simulink model "OLDip_RMS_testOLD"  (R2022b)
settings: Solver=FixedStepAuto  StartTime=0.0  StopTime=inf  FixedStep=Ts  RelTol=1e-3
undefined symbols (not defined in the file or in its folder): countsPerRev, maxPWM, motorN, pendDwnValue, Ts
libraries: arduinolib x6, slpidlib x3, arduinosensorlib x1, hdlsllib x1
settings Model: SimulationMode=external  ExtModeTrigDuration=2  Creator=47954  LastModifiedBy=47954
settings SolverCC: AutoInsertRateTranBlk=on
settings OptimizationCC: EnhancedBackFolding=on  PassReuseOutputArgsThreshold=0  MaxStackSize=64  OptimizeBlockOrder=speed  DifferentSizesBufferReuse=on  OptimizationCustomize=off
settings DebuggingCC: ParameterPrecisionLossMsg=none  ParameterTunabilityLossMsg=error
settings HardwareCC: ProdBitPerInt=16  ProdBitPerPointer=16  ProdBitPerSizeT=16  ProdBitPerPtrDiffT=16  ProdLargestAtomicFloat=None  ProdWordSize=8  ProdLongLongMode=on  ProdHWDeviceType=Atmel->AVR  UseEmbeddedCoderFeatures=off  UseSimulinkCoderFeatures=off
settings ModelReferenceCC: EnableRefExpFcnMdlSchedulingChecks=on
settings SFSimCC: MATLABDynamicMemAlloc=off
settings RTWCC: Description=Embedded Coder  SystemTargetFile=ert.tlc  HardwareBoard=Arduino Mega 2560  TemplateMakefile=ert_default_tmf  RTWVerbose=off  Toolchain=Arduino AVR
settings CodeAppCC: ForceParamTrailComments=on  OperatorAnnotations=on  MangleLength=10
settings ERTTargetCC: ERTCustomFileBanners=off  SupportContinuousTime=on  SupportNonInlinedSFcns=on  RemoveResetFunc=off  SupportVariableSizeSignals=on  ModelStepFunctionPrototypeControlCompliant=off  ExtMode=on  ExtModeTransport=3  ExtModeStaticAlloc=on  ExtModeStaticAllocSize=2048  ExtModeMexFile=ext_xcp  ExtModeMexArgs=0 6 921600  ExtModeIntrfLevel=Level2 - Open  ERTSrcFileBannerTemplate=codertarget_code_template.cgt  ERTHdrFileBannerTemplate=codertarget_code_template.cgt  ERTDataSrcFileTemplate=codertarget_code_template.cgt  ERTDataHdrFileTemplate=codertarget_code_template.cgt

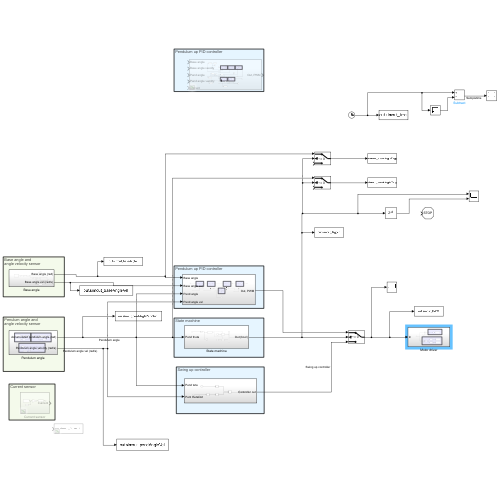
[thumbnail: Simulink's stored preview of the top-level diagram]
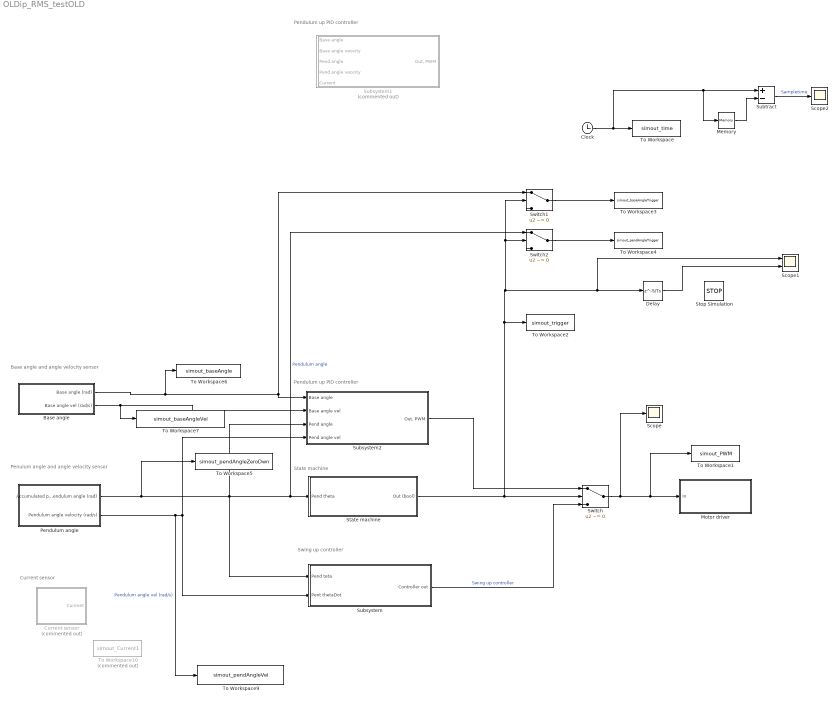
== system OLDip_RMS_testOLD ==
  note: State machine
  note: Swing up controller
  note: Penulum angle and
      | angle velocity sensor
  note: Base angle and
      | angle velocity sensor
  note: Current sensor
  note: Pendulum up PID controller
  note: Pendulum up PID controller
  Base angle : Subsystem
  Clock : Clock
  Current sensor : Subsystem  Commented=on
  Delay : Delay  DelayLength=5/Ts
  Memory : Memory
  Motor driver : Subsystem
  Pendulum angle : Subsystem
  Scope : Scope
  Scope1 : Scope  NumInputPorts=2
  Scope2 : Scope
  State machine : Subsystem
  Stop Simulation : Stop
  Subsystem : Subsystem
  Subsystem1 : Subsystem  Commented=on
  Subsystem2 : Subsystem
  Subtract : Sum  Inputs=+-
  Switch : Switch  Criteria=u2 ~= 0  SaturateOnIntegerOverflow=off  InputSameDT=off
  Switch1 : Switch  Criteria=u2 ~= 0  SaturateOnIntegerOverflow=off  InputSameDT=off
  Switch2 : Switch  Criteria=u2 ~= 0  SaturateOnIntegerOverflow=off  InputSameDT=off
  To Workspace : ToWorkspace  VariableName=simout_time  SampleTime=-1
      settings: Save2DSignal=2-D array (concatenate along first dimension)
  To Workspace1 : ToWorkspace  VariableName=simout_PWM  SampleTime=-1
      settings: Save2DSignal=2-D array (concatenate along first dimension)
  To Workspace10 : ToWorkspace  Commented=on  VariableName=simout_Current1  SampleTime=-1
      settings: Save2DSignal=2-D array (concatenate along first dimension)
  To Workspace2 : ToWorkspace  VariableName=simout_trigger  SampleTime=-1
      settings: Save2DSignal=2-D array (concatenate along first dimension)
  To Workspace3 : ToWorkspace  VariableName=simout_baseAngleTrigger  SampleTime=-1
      settings: Save2DSignal=2-D array (concatenate along first dimension)
  To Workspace4 : ToWorkspace  VariableName=simout_pendAngleTrigger  SampleTime=-1
      settings: Save2DSignal=2-D array (concatenate along first dimension)
  To Workspace5 : ToWorkspace  VariableName=simout_pendAngleZeroDwn  SampleTime=-1
      settings: Save2DSignal=2-D array (concatenate along first dimension)
  To Workspace6 : ToWorkspace  VariableName=simout_baseAngle  SampleTime=-1
      settings: Save2DSignal=2-D array (concatenate along first dimension)
  To Workspace7 : ToWorkspace  VariableName=simout_baseAngleVel  SampleTime=-1
      settings: Save2DSignal=2-D array (concatenate along first dimension)
  To Workspace9 : ToWorkspace  VariableName=simout_pendAngleVel  SampleTime=-1
      settings: Save2DSignal=2-D array (concatenate along first dimension)
  wires:
  Pendulum angle/1(Accumulated pendulum angle (rad)) -> To Workspace5/1, State machine/1(Pend theta), Switch2/1, Subsystem2/3(Pend angle), Subsystem/1(Pend teta)  "Pendulum angle"
  State machine/1(Out (bool)) -> Switch2/2, Switch1/2, Delay/1, Scope1/1, To Workspace2/1, Switch/2
  Subsystem/1(Controller out) -> Switch/3  "Swing up controller"
  Pendulum angle/2(Pendulum angle velocity (rad/s)) -> To Workspace9/1, Subsystem2/4(Pend angle vel), Subsystem/2(Pent thetaDot)  "Pendulum angle vel (rad/s)"
  Subsystem2/1("Out, PWM") -> Switch/1
  Base angle/1(Base angle (rad)) -> To Workspace6/1, Subsystem2/1(Base angle), Switch1/1
  Base angle/2(Base angle vel (rad/s)) -> To Workspace7/1, Subsystem2/2(Base angle vel)
  Switch/1 -> Scope/1, To Workspace1/1, Motor driver/1(In)
  Delay/1 -> Scope1/2
  Switch1/1 -> To Workspace3/1
  Switch2/1 -> To Workspace4/1
  Clock/1 -> Memory/1, Subtract/1, To Workspace/1
  Subtract/1 -> Scope2/1  "Sampletime"
  Memory/1 -> Subtract/2

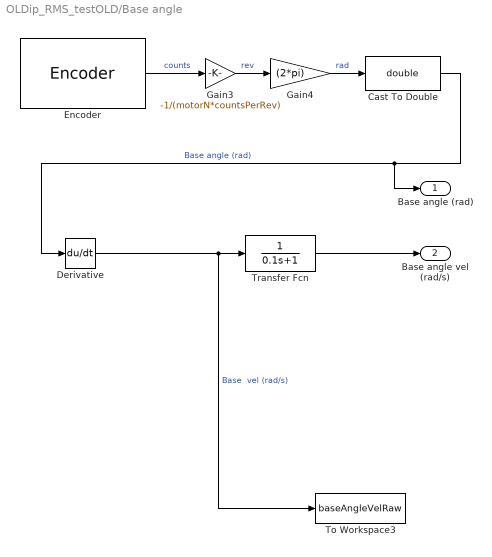
== system OLDip_RMS_testOLD/Base angle ==
  Cast To Double : DataTypeConversion  OutDataTypeStr=double  SaturateOnIntegerOverflow=off  RndMeth=Floor
  Derivative : Derivative
  Encoder : arduinosensorlib/Encoder  InputA=2  InputB=3  Mode=No reset  SampleTime=-1
  Gain3 : Gain  Gain=-1/(motorN*countsPerRev)
  Gain4 : Gain  Gain=(2*pi)
  To Workspace3 : ToWorkspace  VariableName=baseAngleVelRaw  SaveFormat=Structure With Time  SampleTime=-1
      settings: Save2DSignal=2-D array (concatenate along first dimension)
  Transfer Fcn : TransferFcn  Denominator=[0.1 1]
  Base angle (rad) : Outport
  Base angle vel (rad/s) : Outport  Port=2
  wires:
  Gain3/1 -> Gain4/1  "rev"
  Gain4/1 -> Cast To Double/1  "rad"
  Encoder/1 -> Gain3/1  "counts"
  Transfer Fcn/1 -> Base angle vel (rad/s)/1
  Derivative/1 -> To Workspace3/1, Transfer Fcn/1  "Base  vel (rad/s)"
  Cast To Double/1 -> Derivative/1, Base angle (rad)/1  "Base angle (rad)"

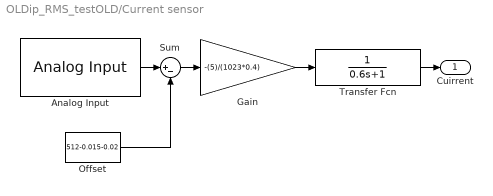
== system OLDip_RMS_testOLD/Current sensor ==
  Analog Input : arduinolib/Analog Input  pinNumber=10  ReadResultsOnly=off  ConversionTriggerSource=Software  ExternalTriggerType=uint32( 0 )  OutputDataType=uint16  EnableConversionCompleteNotify=off  EnableOuputStatus=off  SampleTime=-1  blockPlatform=arduino
  Gain : Gain  Gain=-(5)/(1023*0.4)
  Offset : Constant  Value=512-0.015-0.02
  Sum : Sum  Inputs=|+-
  Transfer Fcn : TransferFcn  Denominator=[0.6 1]
  Cuirrent : Outport
  wires:
  Offset/1 -> Sum/2
  Analog Input/1 -> Sum/1
  Gain/1 -> Transfer Fcn/1
  Transfer Fcn/1 -> Cuirrent/1
  Sum/1 -> Gain/1

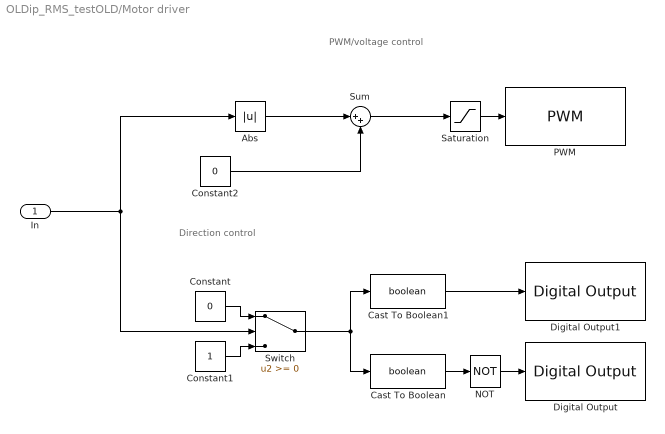
== system OLDip_RMS_testOLD/Motor driver ==
  note: PWM/voltage control
  note: Direction control
  In : Inport
  Abs : Abs  SaturateOnIntegerOverflow=off
  Cast To Boolean : DataTypeConversion  OutDataTypeStr=boolean  SaturateOnIntegerOverflow=off  RndMeth=Floor
  Cast To Boolean1 : DataTypeConversion  OutDataTypeStr=boolean  SaturateOnIntegerOverflow=off  RndMeth=Floor
  Constant : Constant  Value=0
  Constant1 : Constant
  Constant2 : Constant  Value=0
  Digital Output : arduinolib/Digital Output  pinNumber=4  Direction=output  blockPlatform=arduino
  Digital Output1 : arduinolib/Digital Output  pinNumber=5  Direction=output  blockPlatform=arduino
  NOT : Logic  Operator=NOT  IconShape=distinctive  AllPortsSameDT=off  OutDataTypeStr=boolean
  PWM : arduinolib/PWM  pinNumber=13  frequencyType=Specify  desiredFrequency=490.2*2  achievableFrequency=980.4
  Saturation : Saturate  UpperLimit=maxPWM  LowerLimit=-maxPWM
  Sum : Sum  Inputs=|++
  Switch : Switch  SaturateOnIntegerOverflow=off  InputSameDT=off
  wires:
  Constant1/1 -> Switch/3
  Cast To Boolean1/1 -> Digital Output1/1
  Constant/1 -> Switch/1
  In/1 -> Switch/2, Abs/1
  Switch/1 -> Cast To Boolean/1, Cast To Boolean1/1
  Cast To Boolean/1 -> NOT/1
  NOT/1 -> Digital Output/1
  Saturation/1 -> PWM/1
  Abs/1 -> Sum/1
  Sum/1 -> Saturation/1
  Constant2/1 -> Sum/2

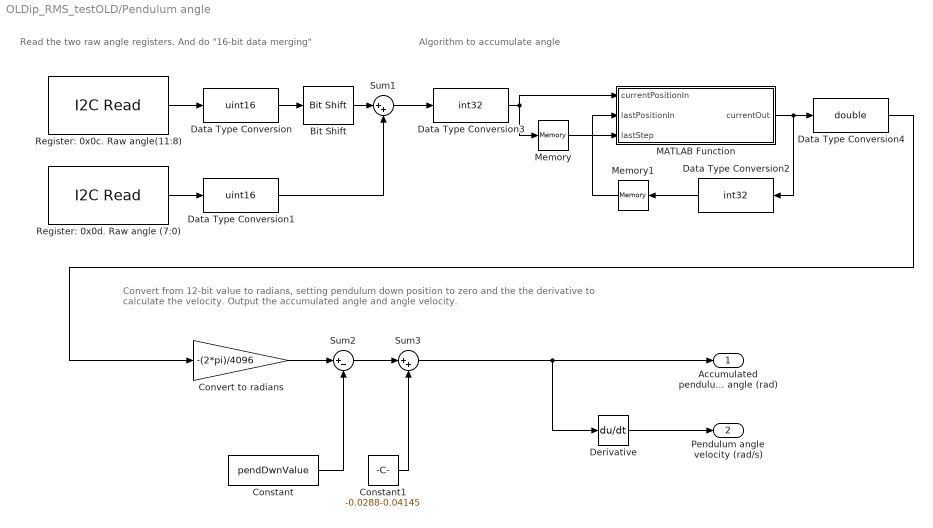
== system OLDip_RMS_testOLD/Pendulum angle ==
  note: Algorithm to accumulate angle
  note: Read the two raw angle registers.
      | And do "16-bit data merging"
  note: Convert from 12-bit value to radians, setting pendulum down position to zero and the the derivative
      | to calculate the velocity. Output the accumulated angle and angle velocity.
  Bit Shift : hdlsllib/Logic and Bit Operations/Bit Shift  mode=Shift Left Logical  N=8
  Constant : Constant  Value=pendDwnValue
  Constant1 : Constant  Value=-0.0288-0.04145
  Convert to radians : Gain  Gain=-(2*pi)/4096
  Data Type Conversion : DataTypeConversion  OutDataTypeStr=uint16  SaturateOnIntegerOverflow=off  RndMeth=Floor
  Data Type Conversion1 : DataTypeConversion  OutDataTypeStr=uint16  SaturateOnIntegerOverflow=off  RndMeth=Floor
  Data Type Conversion2 : DataTypeConversion  OutDataTypeStr=int32  SaturateOnIntegerOverflow=off  RndMeth=Floor
  Data Type Conversion3 : DataTypeConversion  OutDataTypeStr=int32  SaturateOnIntegerOverflow=off  RndMeth=Floor
  Data Type Conversion4 : DataTypeConversion  OutDataTypeStr=double  SaturateOnIntegerOverflow=off  RndMeth=Floor
  Derivative : Derivative
  "MATLAB Function " : MATLAB Function  TreatAsAtomicUnit=on
  Memory : Memory
  Memory1 : Memory
  Register: 0x0c. Raw angle(11:8) : arduinolib/I2C Read  I2CModule=0  Mode=Master  SlaveAddress=0x36  SlaveByteOrder=BigEndian  Direction=Receiver  RegisterAddressMode=on  RegisterAddress=0x0c  SlaveDataType=uint8  DataLength=1  NoAck=off  RepeatedStart=off  OutputStatus=off  blockPlatform=ARDUINO  SampleTime=-1
  Register: 0x0d. Raw angle (7:0) : arduinolib/I2C Read  I2CModule=0  Mode=Master  SlaveAddress=0x36  SlaveByteOrder=BigEndian  Direction=Receiver  RegisterAddressMode=on  RegisterAddress=0x0d  SlaveDataType=uint8  DataLength=1  NoAck=off  RepeatedStart=off  OutputStatus=off  blockPlatform=ARDUINO  SampleTime=-1
  Sum1 : Sum  Inputs=|++
  Sum2 : Sum  Inputs=|+-
  Sum3 : Sum  Inputs=|++
  Accumulated pendulum angle (rad) : Outport
  Pendulum angle velocity (rad/s) : Outport  Port=2
  wires:
  Memory/1 -> "MATLAB Function "/3(lastStep)
  Register: 0x0c. Raw angle(11:8)/1 -> Data Type Conversion/1
  Data Type Conversion3/1 -> Memory/1, "MATLAB Function "/1(currentPositionIn)
  Sum1/1 -> Data Type Conversion3/1
  Register: 0x0d. Raw angle (7:0)/1 -> Data Type Conversion1/1
  Bit Shift/1 -> Sum1/1
  Memory1/1 -> "MATLAB Function "/2(lastPositionIn)
  Data Type Conversion1/1 -> Sum1/2
  Data Type Conversion/1 -> Bit Shift/1
  "MATLAB Function "/1(currentOut) -> Data Type Conversion4/1, Data Type Conversion2/1
  Data Type Conversion2/1 -> Memory1/1
  Data Type Conversion4/1 -> Convert to radians/1
  Convert to radians/1 -> Sum2/1
  Sum3/1 -> Accumulated pendulum angle (rad)/1, Derivative/1
  Derivative/1 -> Pendulum angle velocity (rad/s)/1
  Constant/1 -> Sum2/2
  Constant1/1 -> Sum3/2
  Sum2/1 -> Sum3/1

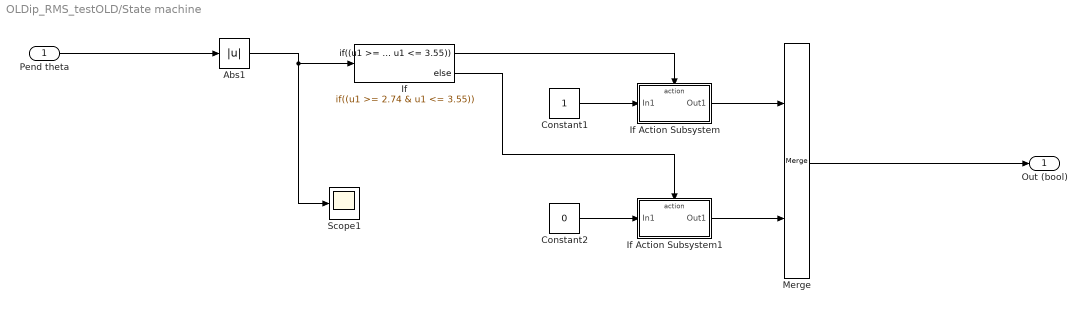
== system OLDip_RMS_testOLD/State machine ==
  Pend theta : Inport
  Abs1 : Abs  SaturateOnIntegerOverflow=off
  Constant1 : Constant
  Constant2 : Constant  Value=0
  If : If  IfExpression=(u1 >= 2.74 & u1 <= 3.55)
  If Action Subsystem : Subsystem  TreatAsAtomicUnit=on
  If Action Subsystem1 : Subsystem  TreatAsAtomicUnit=on
  Merge : Merge
  Scope1 : Scope
  Out (bool) : Outport
  wires:
  Constant1/1 -> If Action Subsystem/1(In1)
  If Action Subsystem/1(Out1) -> Merge/1
  If/1 -> If Action Subsystem/Action
  Pend theta/1 -> Abs1/1
  If/2 -> If Action Subsystem1/Action
  If Action Subsystem1/1(Out1) -> Merge/2
  Constant2/1 -> If Action Subsystem1/1(In1)
  Abs1/1 -> Scope1/1, If/1
  Merge/1 -> Out (bool)/1

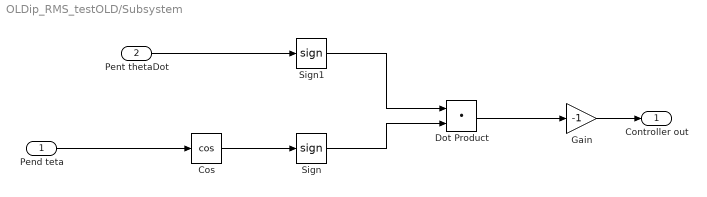
== system OLDip_RMS_testOLD/Subsystem ==
  Pend teta : Inport
  Pent thetaDot : Inport  Port=2
  Cos : Trigonometry  Operator=cos
  Dot Product : DotProduct  OutDataTypeStr=Inherit: Inherit via internal rule
  Gain : Gain  Gain=-1
  Sign : Signum
  Sign1 : Signum
  Controller out : Outport
  wires:
  Pend teta/1 -> Cos/1
  Sign1/1 -> Dot Product/1
  Pent thetaDot/1 -> Sign1/1
  Dot Product/1 -> Gain/1
  Sign/1 -> Dot Product/2
  Cos/1 -> Sign/1
  Gain/1 -> Controller out/1

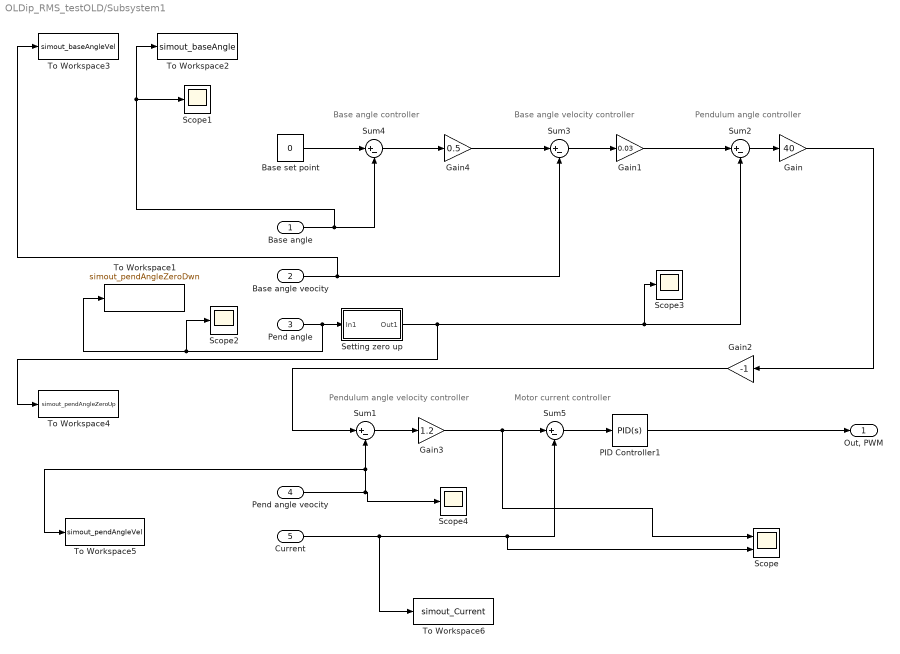
== system OLDip_RMS_testOLD/Subsystem1 ==
  note: Pendulum angle velocity controller
  note: Pendulum angle controller
  note: Base angle velocity controller
  note: Base angle controller
  note: Motor current controller
  Base angle : Inport
  Base angle veocity : Inport  Port=2
  Pend angle : Inport  Port=3
  Pend angle veocity : Inport  Port=4
  Current : Inport  Port=5
  Base set point : Constant  Value=0
  Gain : Gain  Gain=40
  Gain1 : Gain  Gain=0.03
  Gain2 : Gain  Gain=-1
  Gain3 : Gain  Gain=1.2
  Gain4 : Gain  Gain=0.5
  PID Controller1 : slpidlib/PID Controller  Controller=PID  Form=Parallel  TimeDomain=Continuous-time  UseExternalTs=off  SampleTime=-1  IntegratorMethod=Forward Euler  FilterMethod=Forward Euler  ControllerParametersSource=internal  P=30  I=0  UseKiTs=off  D=0  N=100  UseFilter=on  TunerSelectOption=Transfer Function Based (PID Tuner App)  InitialConditionSource=internal  InitialConditionForIntegrator=0  InitialConditionForFilter=0  DifferentiatorICPrevScaledInput=0  ExternalReset=none  TrackingMode=off  Kt=1  LimitOutput=off  SatLimitsSource=internal  UpperSaturationLimit=6  LowerSaturationLimit=-6  LinearizeAsGain=on  AntiWindupMode=clamping  Kb=1  LimitIntegrator=off  UpperIntegratorSaturationLimit=inf  LowerIntegratorSaturationLimit=-inf  POutMin=[]  POutMax=[]  IOutMin=[]  IOutMax=[]  DOutMin=[]  DOutMax=[]  NOutMin=[]  NOutMax=[]  SumOutMin=[]  SumOutMax=[]  SaturationOutMin=[]  SaturationOutMax=[]  PParamMin=[]  PParamMax=[]  IParamMin=[]  IParamMax=[]  DParamMin=[]  DParamMax=[]  NParamMin=[]  NParamMax=[]  KbParamMin=[]  KbParamMax=[]  KtParamMin=[]  KtParamMax=[]  KbOutMin=[]  KbOutMax=[]  KtOutMin=[]  KtOutMax=[]  IntegratorOutMin=[]  IntegratorOutMax=[]  FilterOutMin=[]  FilterOutMax=[]  SumI1OutMin=[]  SumI1OutMax=[]  SumI2OutMin=[]  SumI2OutMax=[]  SumI3OutMin=[]  SumI3OutMax=[]  SumI4OutMin=[]  SumI4OutMax=[]  SumDOutMin=[]  SumDOutMax=[]  DifferentiatorOutMin=[]  DifferentiatorOutMax=[]  FilterDiffOutCoefMin=[]  FilterDiffOutCoefMax=[]  ReciprocalOutMin=[]  ReciprocalOutMax=[]  SumDenOutMin=[]  SumDenOutMax=[]  SumNumOutMin=[]  SumNumOutMax=[]  DivideOutMin=[]  DivideOutMax=[]  UdiffTsProdOutMin=[]  UdiffTsProdOutMax=[]  NTsProdOutMin=[]  NTsProdOutMax=[]  UintegralTsProdOutMin=[]  UintegralTsProdOutMax=[]  UngainTsProdOutMin=[]  UngainTsProdOutMax=[]  ClampingZeroOutDataTypeStr=Inherit: Inherit via back propagation  ClampingZeroOutMin=[]  ClampingZeroOutMax=[]  FilterDenConstantOutDataTypeStr=Inherit: Inherit via back propagation  FilterDenConstantOutMin=[]  FilterDenConstantOutMax=[]  PCopyOutDataTypeStr=Inherit: Inherit via back propagation  PCopyOutMin=[]  PCopyOutMax=[]  NCopyOutDataTypeStr=Inherit: Inherit via back propagation  NCopyOutMin=[]  NCopyOutMax=[]  IntegratorContinuousStateAttributes=''  IntegratorStateMustResolveToSignalObject=off  IntegratorRTWStateStorageClass=Auto  FilterContinuousStateAttributes=''  FilterStateMustResolveToSignalObject=off  FilterRTWStateStorageClass=Auto  ParallelPVariant=InternalParameters  IdealPVariant=Disabled  IVariant=InternalParameters  DVariant=InternalParameters  IntegratorVariant=Continuous  SatVariant=Disabled  AWVariant=Passthrough  PCopyVariant=Disabled  TRVariant=Disabled  FdbkBlocksVariant=Forward  IdealPFdbkVariant=Disabled  SatFdbkVariant=Disabled  DerivativeFilterVariant=ContFilter  NVariant=InternalParameters  NCopyVariant=Disabled  FilterICVariant=InternalICsFilter  IntegratorICVariant=InternalICs  ExternalResetVariant=Disabled  TRSumVariant=Passthrough  SumFdbkVariant=Disabled  SumVariant=Sum_PID  TsampFilterVariant=InternalTs  TsampNgainVariant=Passthrough  TsampIntegralVariant=Passthrough  ExternalSaturationOutDataTypeStr=Inherit: Same as second input
  Scope : Scope  NumInputPorts=2
  Scope{1..4} (4 alike) : Scope
  "Setting zero up " : Subsystem
  Sum{1..5} (5 alike) : Sum  Inputs=|+-
  To Workspace1 : ToWorkspace  VariableName=simout_pendAngleZeroDwn  SampleTime=-1
      settings: Save2DSignal=2-D array (concatenate along first dimension)
  To Workspace2 : ToWorkspace  VariableName=simout_baseAngle  SampleTime=-1
      settings: Save2DSignal=2-D array (concatenate along first dimension)
  To Workspace3 : ToWorkspace  VariableName=simout_baseAngleVel  SampleTime=-1
      settings: Save2DSignal=2-D array (concatenate along first dimension)
  To Workspace4 : ToWorkspace  VariableName=simout_pendAngleZeroUp  SampleTime=-1
      settings: Save2DSignal=2-D array (concatenate along first dimension)
  To Workspace5 : ToWorkspace  VariableName=simout_pendAngleVel  SampleTime=-1
      settings: Save2DSignal=2-D array (concatenate along first dimension)
  To Workspace6 : ToWorkspace  VariableName=simout_Current  SampleTime=-1
      settings: Save2DSignal=2-D array (concatenate along first dimension)
  "Out, PWM" : Outport
  wires:
  Sum2/1 -> Gain/1
  Sum1/1 -> Gain3/1
  Gain/1 -> Gain2/1
  Pend angle veocity/1 -> Scope4/1, To Workspace5/1, Sum1/2
  Sum4/1 -> Gain4/1
  Sum3/1 -> Gain1/1
  Gain1/1 -> Sum2/1
  Gain2/1 -> Sum1/1
  Base angle/1 -> Scope1/1, To Workspace2/1, Sum4/2
  Gain4/1 -> Sum3/1
  Base set point/1 -> Sum4/1
  Sum5/1 -> PID Controller1/1
  Gain3/1 -> Scope/1, Sum5/1
  PID Controller1/1 -> "Out, PWM"/1
  Current/1 -> To Workspace6/1, Scope/2, Sum5/2
  Pend angle/1 -> Scope2/1, To Workspace1/1, "Setting zero up "/1(In1)
  "Setting zero up "/1(Out1) -> To Workspace4/1, Scope3/1, Sum2/2
  Base angle veocity/1 -> To Workspace3/1, Sum3/2

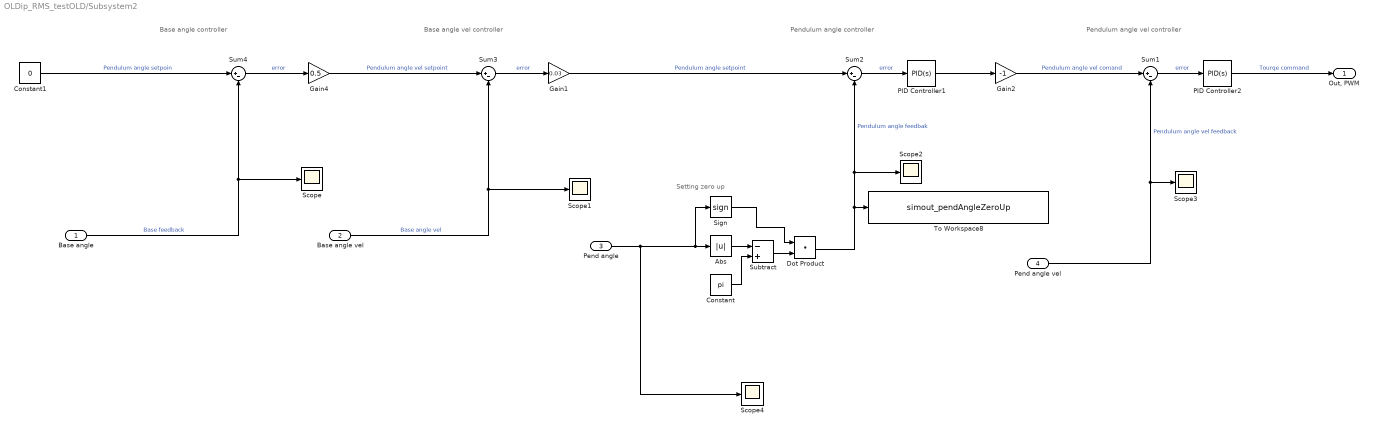
== system OLDip_RMS_testOLD/Subsystem2 ==
  note: Setting zero up
  note: Pendulum angle controller
  note: Pendulum angle vel controller
  note: Base angle vel controller
  note: Base angle controller
  Base angle : Inport
  Base angle vel : Inport  Port=2
  Pend angle : Inport  Port=3
  Pend angle vel : Inport  Port=4
  Abs : Abs  SaturateOnIntegerOverflow=off
  Constant : Constant  Value=pi
  Constant1 : Constant  Value=0
  Dot Product : DotProduct  OutDataTypeStr=Inherit: Inherit via internal rule
  Gain1 : Gain  Gain=0.03
  Gain2 : Gain  Gain=-1
  Gain4 : Gain  Gain=0.5
  PID Controller1 : slpidlib/PID Controller  Controller=PID  Form=Parallel  TimeDomain=Continuous-time  UseExternalTs=off  SampleTime=-1  IntegratorMethod=Forward Euler  FilterMethod=Forward Euler  ControllerParametersSource=internal  P=45  I=0  UseKiTs=off  D=0  N=100  UseFilter=on  TunerSelectOption=Transfer Function Based (PID Tuner App)  InitialConditionSource=internal  InitialConditionForIntegrator=0  InitialConditionForFilter=0  DifferentiatorICPrevScaledInput=0  ExternalReset=none  TrackingMode=off  Kt=1  LimitOutput=off  SatLimitsSource=internal  UpperSaturationLimit=6  LowerSaturationLimit=-6  LinearizeAsGain=on  AntiWindupMode=clamping  Kb=1  LimitIntegrator=off  UpperIntegratorSaturationLimit=inf  LowerIntegratorSaturationLimit=-inf  POutMin=[]  POutMax=[]  IOutMin=[]  IOutMax=[]  DOutMin=[]  DOutMax=[]  NOutMin=[]  NOutMax=[]  SumOutMin=[]  SumOutMax=[]  SaturationOutMin=[]  SaturationOutMax=[]  PParamMin=[]  PParamMax=[]  IParamMin=[]  IParamMax=[]  DParamMin=[]  DParamMax=[]  NParamMin=[]  NParamMax=[]  KbParamMin=[]  KbParamMax=[]  KtParamMin=[]  KtParamMax=[]  KbOutMin=[]  KbOutMax=[]  KtOutMin=[]  KtOutMax=[]  IntegratorOutMin=[]  IntegratorOutMax=[]  FilterOutMin=[]  FilterOutMax=[]  SumI1OutMin=[]  SumI1OutMax=[]  SumI2OutMin=[]  SumI2OutMax=[]  SumI3OutMin=[]  SumI3OutMax=[]  SumI4OutMin=[]  SumI4OutMax=[]  SumDOutMin=[]  SumDOutMax=[]  DifferentiatorOutMin=[]  DifferentiatorOutMax=[]  FilterDiffOutCoefMin=[]  FilterDiffOutCoefMax=[]  ReciprocalOutMin=[]  ReciprocalOutMax=[]  SumDenOutMin=[]  SumDenOutMax=[]  SumNumOutMin=[]  SumNumOutMax=[]  DivideOutMin=[]  DivideOutMax=[]  UdiffTsProdOutMin=[]  UdiffTsProdOutMax=[]  NTsProdOutMin=[]  NTsProdOutMax=[]  UintegralTsProdOutMin=[]  UintegralTsProdOutMax=[]  UngainTsProdOutMin=[]  UngainTsProdOutMax=[]  ClampingZeroOutDataTypeStr=Inherit: Inherit via back propagation  ClampingZeroOutMin=[]  ClampingZeroOutMax=[]  FilterDenConstantOutDataTypeStr=Inherit: Inherit via back propagation  FilterDenConstantOutMin=[]  FilterDenConstantOutMax=[]  PCopyOutDataTypeStr=Inherit: Inherit via back propagation  PCopyOutMin=[]  PCopyOutMax=[]  NCopyOutDataTypeStr=Inherit: Inherit via back propagation  NCopyOutMin=[]  NCopyOutMax=[]  IntegratorContinuousStateAttributes=''  IntegratorStateMustResolveToSignalObject=off  IntegratorRTWStateStorageClass=Auto  FilterContinuousStateAttributes=''  FilterStateMustResolveToSignalObject=off  FilterRTWStateStorageClass=Auto  ParallelPVariant=InternalParameters  IdealPVariant=Disabled  IVariant=InternalParameters  DVariant=InternalParameters  IntegratorVariant=Continuous  SatVariant=Disabled  AWVariant=Passthrough  PCopyVariant=Disabled  TRVariant=Disabled  FdbkBlocksVariant=Forward  IdealPFdbkVariant=Disabled  SatFdbkVariant=Disabled  DerivativeFilterVariant=ContFilter  NVariant=InternalParameters  NCopyVariant=Disabled  FilterICVariant=InternalICsFilter  IntegratorICVariant=InternalICs  ExternalResetVariant=Disabled  TRSumVariant=Passthrough  SumFdbkVariant=Disabled  SumVariant=Sum_PID  TsampFilterVariant=InternalTs  TsampNgainVariant=Passthrough  TsampIntegralVariant=Passthrough  ExternalSaturationOutDataTypeStr=Inherit: Same as second input
  PID Controller2 : slpidlib/PID Controller  Controller=PID  Form=Parallel  TimeDomain=Continuous-time  UseExternalTs=off  SampleTime=-1  IntegratorMethod=Forward Euler  FilterMethod=Forward Euler  ControllerParametersSource=internal  P=45  I=0  UseKiTs=off  D=0  N=100  UseFilter=on  TunerSelectOption=Transfer Function Based (PID Tuner App)  InitialConditionSource=internal  InitialConditionForIntegrator=0  InitialConditionForFilter=0  DifferentiatorICPrevScaledInput=0  ExternalReset=none  TrackingMode=off  Kt=1  LimitOutput=off  SatLimitsSource=internal  UpperSaturationLimit=6  LowerSaturationLimit=-6  LinearizeAsGain=on  AntiWindupMode=clamping  Kb=1  LimitIntegrator=off  UpperIntegratorSaturationLimit=inf  LowerIntegratorSaturationLimit=-inf  POutMin=[]  POutMax=[]  IOutMin=[]  IOutMax=[]  DOutMin=[]  DOutMax=[]  NOutMin=[]  NOutMax=[]  SumOutMin=[]  SumOutMax=[]  SaturationOutMin=[]  SaturationOutMax=[]  PParamMin=[]  PParamMax=[]  IParamMin=[]  IParamMax=[]  DParamMin=[]  DParamMax=[]  NParamMin=[]  NParamMax=[]  KbParamMin=[]  KbParamMax=[]  KtParamMin=[]  KtParamMax=[]  KbOutMin=[]  KbOutMax=[]  KtOutMin=[]  KtOutMax=[]  IntegratorOutMin=[]  IntegratorOutMax=[]  FilterOutMin=[]  FilterOutMax=[]  SumI1OutMin=[]  SumI1OutMax=[]  SumI2OutMin=[]  SumI2OutMax=[]  SumI3OutMin=[]  SumI3OutMax=[]  SumI4OutMin=[]  SumI4OutMax=[]  SumDOutMin=[]  SumDOutMax=[]  DifferentiatorOutMin=[]  DifferentiatorOutMax=[]  FilterDiffOutCoefMin=[]  FilterDiffOutCoefMax=[]  ReciprocalOutMin=[]  ReciprocalOutMax=[]  SumDenOutMin=[]  SumDenOutMax=[]  SumNumOutMin=[]  SumNumOutMax=[]  DivideOutMin=[]  DivideOutMax=[]  UdiffTsProdOutMin=[]  UdiffTsProdOutMax=[]  NTsProdOutMin=[]  NTsProdOutMax=[]  UintegralTsProdOutMin=[]  UintegralTsProdOutMax=[]  UngainTsProdOutMin=[]  UngainTsProdOutMax=[]  ClampingZeroOutDataTypeStr=Inherit: Inherit via back propagation  ClampingZeroOutMin=[]  ClampingZeroOutMax=[]  FilterDenConstantOutDataTypeStr=Inherit: Inherit via back propagation  FilterDenConstantOutMin=[]  FilterDenConstantOutMax=[]  PCopyOutDataTypeStr=Inherit: Inherit via back propagation  PCopyOutMin=[]  PCopyOutMax=[]  NCopyOutDataTypeStr=Inherit: Inherit via back propagation  NCopyOutMin=[]  NCopyOutMax=[]  IntegratorContinuousStateAttributes=''  IntegratorStateMustResolveToSignalObject=off  IntegratorRTWStateStorageClass=Auto  FilterContinuousStateAttributes=''  FilterStateMustResolveToSignalObject=off  FilterRTWStateStorageClass=Auto  ParallelPVariant=InternalParameters  IdealPVariant=Disabled  IVariant=InternalParameters  DVariant=InternalParameters  IntegratorVariant=Continuous  SatVariant=Disabled  AWVariant=Passthrough  PCopyVariant=Disabled  TRVariant=Disabled  FdbkBlocksVariant=Forward  IdealPFdbkVariant=Disabled  SatFdbkVariant=Disabled  DerivativeFilterVariant=ContFilter  NVariant=InternalParameters  NCopyVariant=Disabled  FilterICVariant=InternalICsFilter  IntegratorICVariant=InternalICs  ExternalResetVariant=Disabled  TRSumVariant=Passthrough  SumFdbkVariant=Disabled  SumVariant=Sum_PID  TsampFilterVariant=InternalTs  TsampNgainVariant=Passthrough  TsampIntegralVariant=Passthrough  ExternalSaturationOutDataTypeStr=Inherit: Same as second input
  Scope{,1..4} (5 alike) : Scope
  Sign : Signum
  Subtract : Sum  Inputs=-+
  Sum{1..4} (4 alike) : Sum  Inputs=|+-
  To Workspace8 : ToWorkspace  VariableName=simout_pendAngleZeroUp  SampleTime=-1
      settings: Save2DSignal=2-D array (concatenate along first dimension)
  "Out, PWM" : Outport
  wires:
  Sum2/1 -> PID Controller1/1  "error"
  Pend angle/1 -> Scope4/1, Sign/1, Abs/1
  Abs/1 -> Subtract/1
  Constant/1 -> Subtract/2
  Subtract/1 -> Dot Product/2
  Dot Product/1 -> Scope2/1, Sum2/2, To Workspace8/1  "Pendulum angle feedbak"
  Sign/1 -> Dot Product/1
  Sum1/1 -> PID Controller2/1  "error"
  PID Controller1/1 -> Gain2/1
  Pend angle vel/1 -> Scope3/1, Sum1/2  "Pendulum angle vel feedback"
  PID Controller2/1 -> "Out, PWM"/1  "Tourqe command"
  Base angle vel/1 -> Scope1/1, Sum3/2  "Base angle vel"
  Sum4/1 -> Gain4/1  "error"
  Sum3/1 -> Gain1/1  "error"
  Gain1/1 -> Sum2/1  "Pendulum angle setpoint"
  Gain2/1 -> Sum1/1  "Pendulum angle vel comand"
  Base angle/1 -> Scope/1, Sum4/2  "Base feedback"
  Gain4/1 -> Sum3/1  "Pendulum angle vel setpoint"
  Constant1/1 -> Sum4/1  "Pendulum angle setpoin"

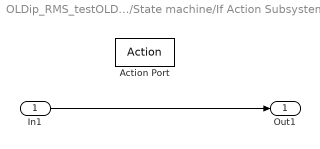
== system OLDip_RMS_testOLD/State machine/If Action Subsystem ==
  In1 : Inport
  Action Port : ActionPort  ActionPortLabel=if((u1 >= 2.74 & u1 <= 3.55))
  Out1 : Outport
  wires:
  In1/1 -> Out1/1

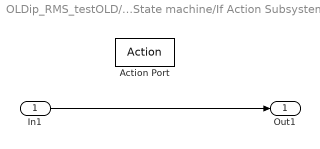
== system OLDip_RMS_testOLD/State machine/If Action Subsystem1 ==
  In1 : Inport
  Action Port : ActionPort  ActionPortLabel=else
  Out1 : Outport
  wires:
  In1/1 -> Out1/1

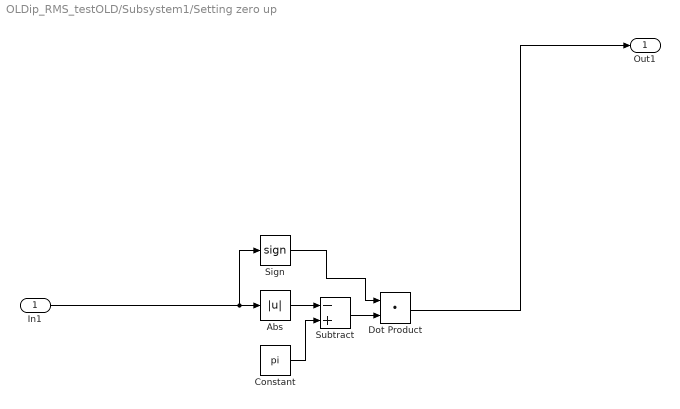
== system OLDip_RMS_testOLD/Subsystem1/Setting zero up  ==
  In1 : Inport
  Abs : Abs  SaturateOnIntegerOverflow=off
  Constant : Constant  Value=pi
  Dot Product : DotProduct  OutDataTypeStr=Inherit: Inherit via internal rule
  Sign : Signum
  Subtract : Sum  Inputs=-+
  Out1 : Outport
  wires:
  Sign/1 -> Dot Product/1
  In1/1 -> Sign/1, Abs/1
  Subtract/1 -> Dot Product/2
  Abs/1 -> Subtract/1
  Constant/1 -> Subtract/2
  Dot Product/1 -> Out1/1

== matlab function OLDip_RMS_testOLD/Pendulum angle/MATLAB Function  ==
  data: currentPositionIn input; currentOut output; lastPositionIn input; lastStep input
function currentOut  = fcn(currentPositionIn, lastPositionIn, lastStep)


if((lastStep > 2048) && (currentPositionIn <(lastStep - 2048)))
    currentOut = lastPositionIn + 4096 - lastStep + currentPositionIn;
elseif((currentPositionIn > 2048) && ( lastStep < (currentPositionIn - 2048)))
    currentOut = lastPositionIn - 4096 - lastStep + currentPositionIn;
else
    currentOut = lastPositionIn - lastStep + currentPositionIn;
end
